simulink model "UT"  (R2022a)
settings: Solver=VariableStepAuto  StartTime=0.0  StopTime=72  RelTol=1e-3
libraries: simulink x1
settings Model: Creator=a.dehghan  LastModifiedBy=a.dehghan

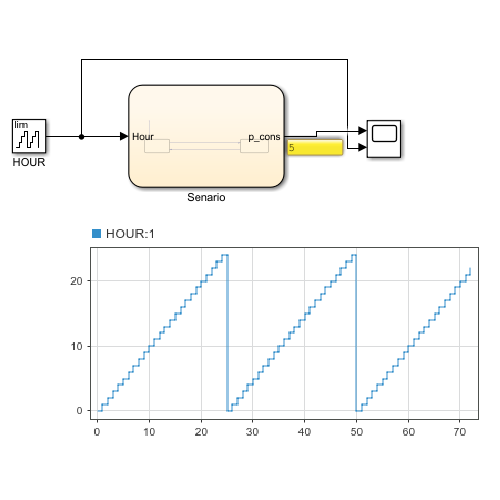
[thumbnail: Simulink's stored preview of the top-level diagram]
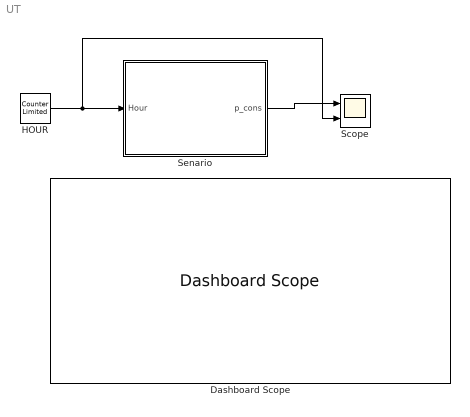
== system UT ==
  Dashboard Scope : DashboardScope
  HOUR : simulink/Sources/Counter Limited  uplimit=24  tsamp=1
  Scope : Scope  NumInputPorts=2
  Senario : Stateflow chart  TreatAsAtomicUnit=on
  wires:
  HOUR/1 -> Scope/2, Senario/1(Hour)
  Senario/1(p_cons) -> Scope/1

== stateflow chart UT/Senario ==
  state decharge
    entry : p_cons = 5;
  state charge
    entry : p_cons = -5
  (default) -> decharge
  decharge -> charge : [Hour >= 12 && Hour < 18]
  charge -> decharge : [Hour >=18]
  data: Hour input; p_cons output
